simulink model "Power_Grid_Fault_Analysis_"  (R2019b)
settings: Solver=FixedStepAuto  StartTime=0.0  StopTime=0.2  RelTol=1e-3
InitFcn:
  | basekV = 23;
  | baseMVA = 100;
  | 
  | % base impedance
  | baseZ = (basekV)^2/baseMVA;
  | 
  | % nominal frequency
  | freq = 50;
libraries: powerlib x64, powerlib_meascontrol x17
(part 2 of 4)

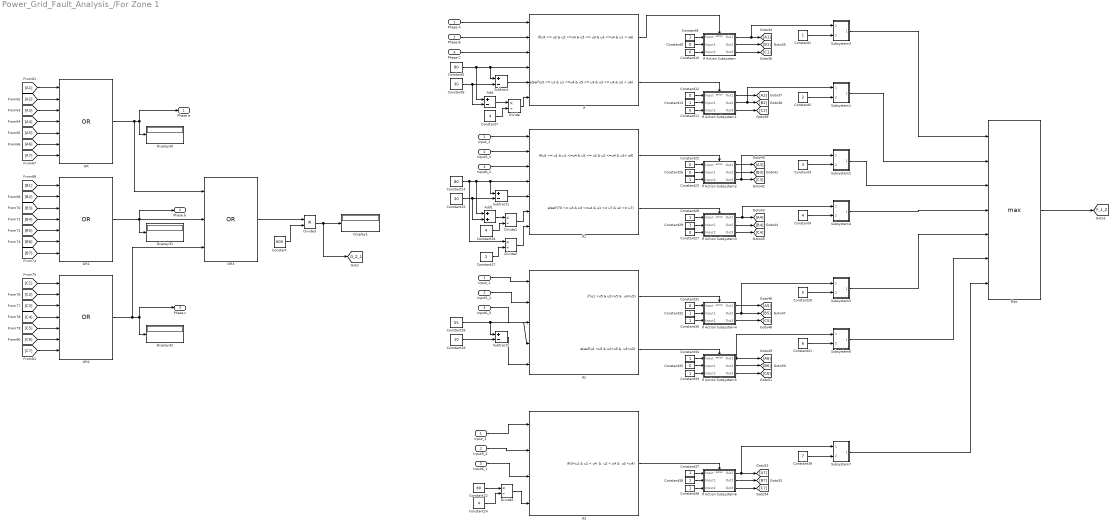
== system Power_Grid_Fault_Analysis_/For Zone 1 ==
  Phase A : Inport
  Phase B : Inport  Port=2
  Phase C : Inport  Port=3
  Add : Sum  Inputs=+-
  Add1 : Sum
  Constant : Constant  Value=600
  Constant{1,8,13,23,28..30,32..34,36..38} (13 alike) : Constant
  Constant{9..12,25..27,31,35} (9 alike) : Constant  Value=0
  Constant14 : Constant  Value=80
  Constant15 : Constant  Value=30
  Constant{4,7,16,24} (4 alike) : Constant  Value=4
  Constant17 : Constant  Value=2
  Constant18 : Constant  Value=55
  Constant19 : Constant  Value=10
  Constant2 : Constant  Value=2
  Constant20 : Constant  Value=5
  Constant21 : Constant  Value=6
  Constant22 : Constant  Value=80
  Constant3 : Constant  Value=3
  Constant39 : Constant  Value=7
  Constant5 : Constant  Value=80
  Constant6 : Constant  Value=30
  Display{1,30..32} (4 alike) : Display
      settings: Decimation=2
  Divide{,1..2,5} (4 alike) : Product  Inputs=*/  SaturateOnIntegerOverflow=on  RndMeth=Zero
  Divide3 : Product  Inputs=**  SaturateOnIntegerOverflow=on  RndMeth=Zero
  If : If  NumInputs=6  IfExpression=u5 <= u2 & u2 <=u4 & u5 <= u3 & u3 <=u4 & u1 < u6  ElseIfExpressions=u5 <= u1 & u1 <=u4 & u5 <= u3 & u3 <= u4 & u2 < u6  ShowElse=off
  If Action Subsystem : Subsystem  TreatAsAtomicUnit=on
  If Action Subsystem1 : Subsystem  TreatAsAtomicUnit=on
  If Action Subsystem2 : Subsystem  TreatAsAtomicUnit=on
  If Action Subsystem3 : Subsystem  TreatAsAtomicUnit=on
  If Action Subsystem4 : Subsystem  TreatAsAtomicUnit=on
  If Action Subsystem5 : Subsystem  TreatAsAtomicUnit=on
  If Action Subsystem6 : Subsystem  TreatAsAtomicUnit=on
  If1 : If  NumInputs=7  IfExpression=u5 <= u1 & u1 <=u4 & u5 <= u2 & u2 <=u4 & u3< u6  ElseIfExpressions=70 <= u3 & u3 <=u4 & u1 <= u7 & u2 <= u7  ShowElse=off
  If2 : If  NumInputs=5  IfExpression="u1 >u5 & u2<u5 &  u3<u5"  ElseIfExpressions="u1 <u5 & u2>u5 &  u3<u5"  ShowElse=off
  If3 : If  NumInputs=4  IfExpression="0<u1 & u1 < u4  &  u2 < u4 &  u3 <u4"  ShowElse=off
  Input5_1 : InportShadow  Port=2
  Input5_2 : InportShadow  Port=2
  Input5_3 : InportShadow  Port=2
  Input6_1 : InportShadow  Port=3
  Input6_2 : InportShadow  Port=3
  Input6_3 : InportShadow  Port=3
  Input_1 : InportShadow
  Input_2 : InportShadow
  Input_3 : InportShadow
  Max : MinMax  Function=max  Inputs=7
  OR : Logic  Operator=OR  Inputs=7  IconShape=distinctive  AllPortsSameDT=off  OutDataTypeStr=boolean
  OR1 : Logic  Operator=OR  Inputs=7  IconShape=distinctive  AllPortsSameDT=off  OutDataTypeStr=boolean
  OR2 : Logic  Operator=OR  Inputs=7  IconShape=distinctive  AllPortsSameDT=off  OutDataTypeStr=boolean
  OR3 : Logic  Operator=OR  Inputs=3  IconShape=distinctive  AllPortsSameDT=off  OutDataTypeStr=boolean
  Subsystem1 : Subsystem
  Subsystem2 : Subsystem
  Subsystem3 : Subsystem
  Subsystem4 : Subsystem
  Subsystem5 : Subsystem
  Subsystem6 : Subsystem
  Subsystem7 : Subsystem
  Subtract : Sum  Inputs=+-
  Subtract1 : Sum  Inputs=+-
  Subtract2 : Sum  Inputs=+-
  Phase a : Outport
  Phase b : Outport  Port=2
  Phase c : Outport  Port=3
  tag scope: D_Z_1=global, F_1_Z=global
  wires:
  If3/1 -> If Action Subsystem6/Action
  Constant5/1 -> Add/1, Subtract/1, If/4
  Constant14/1 -> Divide2/1, Subtract1/1, If1/4, Add1/1
  Constant33/1 -> If Action Subsystem5/3(Input2)
  Subtract/1 -> If/5
  Constant10/1 -> If Action Subsystem/3(Input2)
  Constant6/1 -> Add/2, Subtract/2
  Phase A/1 -> If/1
  Constant9/1 -> If Action Subsystem/2(Input1)
  If2/1 -> If Action Subsystem4/Action
  Constant30/1 -> If Action Subsystem4/3(Input2)
  Input_1/1 -> If2/1
  Input5_1/1 -> If2/2
  If Action Subsystem2/2(Out2) -> [B3]
  Phase B/1 -> If/2
  If2/2 -> If Action Subsystem5/Action
  If Action Subsystem/3(Out3) -> [C1]
  Constant15/1 -> Subtract1/2, Add1/2
  Input5_2/1 -> If3/2
  [A2] -> OR/2
  Input6_3/1 -> If2/3
  If Action Subsystem4/3(Out3) -> [C5]
  If1/1 -> If Action Subsystem2/Action
  Input6_2/1 -> If1/3
  Input_2/1 -> If1/1
  If Action Subsystem1/3(Out3) -> [C2]
  Phase C/1 -> If/3
  Constant24/1 -> Divide5/2
  Subtract2/1 -> If2/5
  Divide2/1 -> If1/7
  Constant18/1 -> Subtract2/1, If2/4
  Constant7/1 -> Divide/2
  Constant8/1 -> If Action Subsystem/1(Input)
  If Action Subsystem6/3(Out3) -> [C7]
  Constant16/1 -> Divide1/2
  If Action Subsystem1/1(Out1) -> [A2]
  Divide/1 -> If/6
  Subtract1/1 -> If1/5
  Constant28/1 -> If Action Subsystem3/1(Input)
  Add1/1 -> Divide1/1
  Constant19/1 -> Subtract2/2
  If/2 -> If Action Subsystem1/Action
  Constant38/1 -> If Action Subsystem6/2(Input1)
  Constant13/1 -> If Action Subsystem1/2(Input1)
  Constant12/1 -> If Action Subsystem1/1(Input)
  If Action Subsystem3/2(Out2) -> [B4]
  Constant17/1 -> Divide2/2
  Constant32/1 -> If Action Subsystem4/2(Input1)
  Constant11/1 -> If Action Subsystem1/3(Input2)
  [A3] -> OR/3
  Constant29/1 -> If Action Subsystem3/2(Input1)
  Constant26/1 -> If Action Subsystem2/2(Input1)
  Add/1 -> Divide/1
  If Action Subsystem3/1(Out1) -> Subsystem4/1(In1), [A4]
  Divide1/1 -> If1/6
  Input_3/1 -> If3/1
  Constant34/1 -> If Action Subsystem5/1(Input)
  Constant27/1 -> If Action Subsystem3/3(Input2)
  Constant25/1 -> If Action Subsystem2/1(Input)
  If/1 -> If Action Subsystem/Action
  Constant22/1 -> Divide5/1
  Constant37/1 -> If Action Subsystem6/1(Input)
  If1/2 -> If Action Subsystem3/Action
  [C4] -> OR2/4
  Divide5/1 -> If3/4
  If Action Subsystem/2(Out2) -> [B1]
  [A1] -> OR/1
  [B5] -> OR1/5
  [B7] -> OR1/7
  [A4] -> OR/4
  If Action Subsystem6/2(Out2) -> [B7]
  [B3] -> OR1/3
  [B6] -> OR1/6
  [B2] -> OR1/2
  If Action Subsystem5/2(Out2) -> [B6]
  If Action Subsystem5/3(Out3) -> [C6]
  [A5] -> OR/5
  [C5] -> OR2/5
  [C1] -> OR2/1
  Constant23/1 -> If Action Subsystem2/3(Input2)
  Constant35/1 -> If Action Subsystem5/2(Input1)
  Input6_1/1 -> If3/3
  [A7] -> OR/7
  [C7] -> OR2/7
  Constant36/1 -> If Action Subsystem6/3(Input2)
  If Action Subsystem4/1(Out1) -> [A5]
  [C3] -> OR2/3
  [B1] -> OR1/1
  [A6] -> OR/6
  Constant31/1 -> If Action Subsystem4/1(Input)
  If Action Subsystem2/1(Out1) -> [A3]
  [C2] -> OR2/2
  [B4] -> OR1/4
  [C6] -> OR2/6
  Input5_3/1 -> If1/2
  Divide3/1 -> [D_Z_1], Display1/1
  OR3/1 -> Divide3/1
  OR2/1 -> OR3/3, Phase c/1, Display32/1
  OR1/1 -> OR3/2, Phase b/1, Display31/1
  Constant/1 -> Divide3/2
  OR/1 -> OR3/1, Phase a/1, Display30/1
  If Action Subsystem/1(Out1) -> Subsystem3/1(In1), [A1]
  Constant1/1 -> Subsystem3/2(In2)
  If Action Subsystem1/2(Out2) -> Subsystem1/1(In1), [B2]
  Constant2/1 -> Subsystem1/2(In2)
  If Action Subsystem2/3(Out3) -> Subsystem2/1(In1), [C3]
  Constant3/1 -> Subsystem2/2(In2)
  Constant4/1 -> Subsystem4/2(In2)
  If Action Subsystem3/3(Out3) -> [C4]
  Constant20/1 -> Subsystem5/2(In2)
  If Action Subsystem4/2(Out2) -> Subsystem5/1(In1), [B5]
  Constant21/1 -> Subsystem6/2(In2)
  If Action Subsystem5/1(Out1) -> Subsystem6/1(In1), [A6]
  Constant39/1 -> Subsystem7/2(In2)
  If Action Subsystem6/1(Out1) -> Subsystem7/1(In1), [A7]
  Subsystem3/1(Output) -> Max/1
  Subsystem1/1(Output) -> Max/2
  Subsystem2/1(Output) -> Max/3
  Subsystem4/1(Output) -> Max/4
  Subsystem5/1(Output) -> Max/5
  Subsystem6/1(Output) -> Max/6
  Subsystem7/1(Output) -> Max/7
  Max/1 -> [F_1_Z]

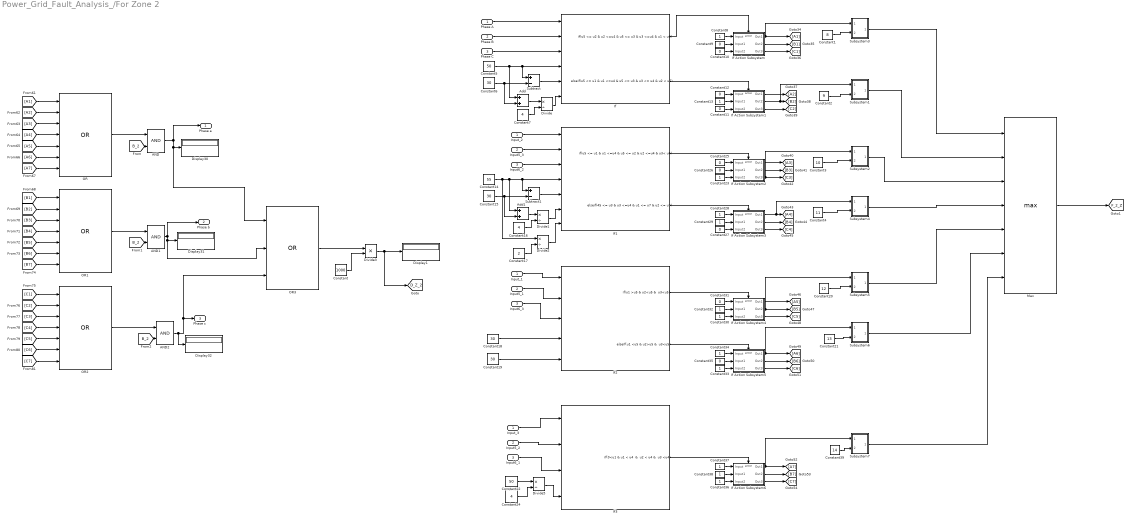
== system Power_Grid_Fault_Analysis_/For Zone 2 ==
  Phase A : Inport
  Phase B : Inport  Port=2
  Phase C : Inport  Port=3
  AND : Logic  IconShape=distinctive  AllPortsSameDT=off  OutDataTypeStr=boolean
  AND1 : Logic  IconShape=distinctive  AllPortsSameDT=off  OutDataTypeStr=boolean
  AND2 : Logic  IconShape=distinctive  AllPortsSameDT=off  OutDataTypeStr=boolean
  Add : Sum
  Add1 : Sum
  Constant : Constant  Value=1000
  Constant1 : Constant  Value=8
  Constant{9..12,25..27,31,35} (9 alike) : Constant  Value=0
  Constant{8,13,23,28..30,32..34,36..38} (12 alike) : Constant
  Constant14 : Constant  Value=55
  Constant{6,15,18..19} (4 alike) : Constant  Value=30
  Constant16 : Constant  Value=4
  Constant17 : Constant  Value=2
  Constant2 : Constant  Value=9
  Constant20 : Constant  Value=12
  Constant21 : Constant  Value=13
  Constant22 : Constant  Value=50
  Constant24 : Constant  Value=4
  Constant3 : Constant  Value=10
  Constant39 : Constant  Value=14
  Constant4 : Constant  Value=11
  Constant5 : Constant  Value=50
  Constant7 : Constant  Value=4
  Display{1,30..32} (4 alike) : Display
      settings: Decimation=2
  Divide{,1..2,5} (4 alike) : Product  Inputs=*/  SaturateOnIntegerOverflow=on  RndMeth=Zero
  Divide3 : Product  Inputs=**  SaturateOnIntegerOverflow=on  RndMeth=Zero
  If : If  NumInputs=6  IfExpression=u5 <= u2 & u2 <=u4 & u5 <= u3 & u3 <=u4 & u1 < u6  ElseIfExpressions=u5 <= u1 & u1 <=u4 & u5 <= u3 & u3 <= u4 & u2 < u6  ShowElse=off
  If Action Subsystem : Subsystem  TreatAsAtomicUnit=on
  If Action Subsystem1 : Subsystem  TreatAsAtomicUnit=on
  If Action Subsystem2 : Subsystem  TreatAsAtomicUnit=on
  If Action Subsystem3 : Subsystem  TreatAsAtomicUnit=on
  If Action Subsystem4 : Subsystem  TreatAsAtomicUnit=on
  If Action Subsystem5 : Subsystem  TreatAsAtomicUnit=on
  If Action Subsystem6 : Subsystem  TreatAsAtomicUnit=on
  If1 : If  NumInputs=7  IfExpression=u5 <= u1 & u1 <=u4 & u5 <= u2 & u2 <=u4 & u3< u6  ElseIfExpressions=45 <= u3 & u3 <=u4 & u1 <= u7 & u2 <= u7  ShowElse=off
  If2 : If  NumInputs=5  IfExpression="u1 >u5 & u2<u5 &  u3<u5"  ElseIfExpressions="u1 <u5 & u2>u5 &  u3<u5"  ShowElse=off
  If3 : If  NumInputs=4  IfExpression="0<u1 & u1 < u4  &  u2 < u4 &  u3 <u4"  ShowElse=off
  Input5_1 : InportShadow  Port=2
  Input5_2 : InportShadow  Port=2
  Input5_3 : InportShadow  Port=2
  Input6_1 : InportShadow  Port=3
  Input6_2 : InportShadow  Port=3
  Input6_3 : InportShadow  Port=3
  Input_1 : InportShadow
  Input_2 : InportShadow
  Input_3 : InportShadow
  Max : MinMax  Function=max  Inputs=7
  OR : Logic  Operator=OR  Inputs=7  IconShape=distinctive  AllPortsSameDT=off  OutDataTypeStr=boolean
  OR1 : Logic  Operator=OR  Inputs=7  IconShape=distinctive  AllPortsSameDT=off  OutDataTypeStr=boolean
  OR2 : Logic  Operator=OR  Inputs=7  IconShape=distinctive  AllPortsSameDT=off  OutDataTypeStr=boolean
  OR3 : Logic  Operator=OR  Inputs=3  IconShape=distinctive  AllPortsSameDT=off  OutDataTypeStr=boolean
  Subsystem1 : Subsystem
  Subsystem2 : Subsystem
  Subsystem3 : Subsystem
  Subsystem4 : Subsystem
  Subsystem5 : Subsystem
  Subsystem6 : Subsystem
  Subsystem7 : Subsystem
  Subtract : Sum  Inputs=+-
  Subtract1 : Sum  Inputs=+-
  Phase a : Outport
  Phase b : Outport  Port=2
  Phase c : Outport  Port=3
  tag scope: D_Z_2=global, F_2_Z=global
  wires:
  If3/1 -> If Action Subsystem6/Action
  Constant5/1 -> Add/1, Subtract/1, If/4
  Constant14/1 -> Divide2/1, Subtract1/1, If1/4, Add1/1
  Constant33/1 -> If Action Subsystem5/3(Input2)
  Subtract/1 -> If/5
  Constant10/1 -> If Action Subsystem/3(Input2)
  Constant6/1 -> Add/2, Subtract/2
  Phase A/1 -> If/1
  Constant9/1 -> If Action Subsystem/2(Input1)
  If2/1 -> If Action Subsystem4/Action
  Constant30/1 -> If Action Subsystem4/3(Input2)
  Input_1/1 -> If2/1
  Input5_1/1 -> If2/2
  If Action Subsystem2/2(Out2) -> [B3]
  Phase B/1 -> If/2
  If2/2 -> If Action Subsystem5/Action
  If Action Subsystem/3(Out3) -> [C1]
  Constant15/1 -> Subtract1/2, Add1/2
  Input5_2/1 -> If3/2
  [A2] -> OR/2
  Input6_3/1 -> If2/3
  If Action Subsystem4/3(Out3) -> [C5]
  If1/1 -> If Action Subsystem2/Action
  Input6_2/1 -> If1/3
  Input_2/1 -> If1/1
  If Action Subsystem1/3(Out3) -> [C2]
  Phase C/1 -> If/3
  Constant24/1 -> Divide5/2
  Constant19/1 -> If2/5
  Divide2/1 -> If1/7
  Constant18/1 -> If2/4
  Constant7/1 -> Divide/2
  Constant8/1 -> If Action Subsystem/1(Input)
  If Action Subsystem6/3(Out3) -> [C7]
  Constant16/1 -> Divide1/2
  If Action Subsystem1/1(Out1) -> [A2]
  Divide/1 -> If/6
  Subtract1/1 -> If1/5
  Constant28/1 -> If Action Subsystem3/1(Input)
  Add1/1 -> Divide1/1
  If/2 -> If Action Subsystem1/Action
  Constant38/1 -> If Action Subsystem6/2(Input1)
  Constant13/1 -> If Action Subsystem1/2(Input1)
  Constant12/1 -> If Action Subsystem1/1(Input)
  If Action Subsystem3/2(Out2) -> [B4]
  Constant17/1 -> Divide2/2
  Constant32/1 -> If Action Subsystem4/2(Input1)
  Constant11/1 -> If Action Subsystem1/3(Input2)
  [A3] -> OR/3
  Constant29/1 -> If Action Subsystem3/2(Input1)
  Constant26/1 -> If Action Subsystem2/2(Input1)
  Add/1 -> Divide/1
  If Action Subsystem3/1(Out1) -> Subsystem4/1(In1), [A4]
  Divide1/1 -> If1/6
  Input_3/1 -> If3/1
  Constant34/1 -> If Action Subsystem5/1(Input)
  Constant27/1 -> If Action Subsystem3/3(Input2)
  Constant25/1 -> If Action Subsystem2/1(Input)
  If/1 -> If Action Subsystem/Action
  Constant22/1 -> Divide5/1
  Constant37/1 -> If Action Subsystem6/1(Input)
  If1/2 -> If Action Subsystem3/Action
  [C4] -> OR2/4
  Divide5/1 -> If3/4
  If Action Subsystem/2(Out2) -> [B1]
  [A1] -> OR/1
  [B5] -> OR1/5
  [B7] -> OR1/7
  [A4] -> OR/4
  If Action Subsystem6/2(Out2) -> [B7]
  [B3] -> OR1/3
  [B6] -> OR1/6
  [B2] -> OR1/2
  If Action Subsystem5/2(Out2) -> [B6]
  If Action Subsystem5/3(Out3) -> [C6]
  [A5] -> OR/5
  [C5] -> OR2/5
  [C1] -> OR2/1
  Constant23/1 -> If Action Subsystem2/3(Input2)
  Constant35/1 -> If Action Subsystem5/2(Input1)
  Input6_1/1 -> If3/3
  [A7] -> OR/7
  [C7] -> OR2/7
  Constant36/1 -> If Action Subsystem6/3(Input2)
  If Action Subsystem4/1(Out1) -> [A5]
  [C3] -> OR2/3
  [B1] -> OR1/1
  [A6] -> OR/6
  Constant31/1 -> If Action Subsystem4/1(Input)
  If Action Subsystem2/1(Out1) -> [A3]
  [C2] -> OR2/2
  [B4] -> OR1/4
  [C6] -> OR2/6
  Input5_3/1 -> If1/2
  Divide3/1 -> [D_Z_2], Display1/1
  OR3/1 -> Divide3/1
  Constant/1 -> Divide3/2
  [B_2] -> AND/2
  OR/1 -> AND/1
  AND/1 -> Phase a/1, OR3/1, Display30/1
  [B_2] -> AND1/2
  OR1/1 -> AND1/1
  AND1/1 -> Phase b/1, OR3/2, Display31/1
  [B_2] -> AND2/2
  OR2/1 -> AND2/1
  AND2/1 -> Display32/1, OR3/3, Phase c/1
  If Action Subsystem6/1(Out1) -> Subsystem7/1(In1), [A7]
  If Action Subsystem/1(Out1) -> Subsystem3/1(In1), [A1]
  If Action Subsystem1/2(Out2) -> Subsystem1/1(In1), [B2]
  Constant20/1 -> Subsystem5/2(In2)
  Constant21/1 -> Subsystem6/2(In2)
  Constant4/1 -> Subsystem4/2(In2)
  Constant39/1 -> Subsystem7/2(In2)
  If Action Subsystem3/3(Out3) -> [C4]
  If Action Subsystem2/3(Out3) -> Subsystem2/1(In1), [C3]
  If Action Subsystem5/1(Out1) -> Subsystem6/1(In1), [A6]
  Constant2/1 -> Subsystem1/2(In2)
  Constant1/1 -> Subsystem3/2(In2)
  If Action Subsystem4/2(Out2) -> Subsystem5/1(In1), [B5]
  Constant3/1 -> Subsystem2/2(In2)
  Subsystem1/1(Output) -> Max/2
  Max/1 -> [F_2_Z]
  Subsystem7/1(Output) -> Max/7
  Subsystem6/1(Output) -> Max/6
  Subsystem5/1(Output) -> Max/5
  Subsystem4/1(Output) -> Max/4
  Subsystem2/1(Output) -> Max/3
  Subsystem3/1(Output) -> Max/1

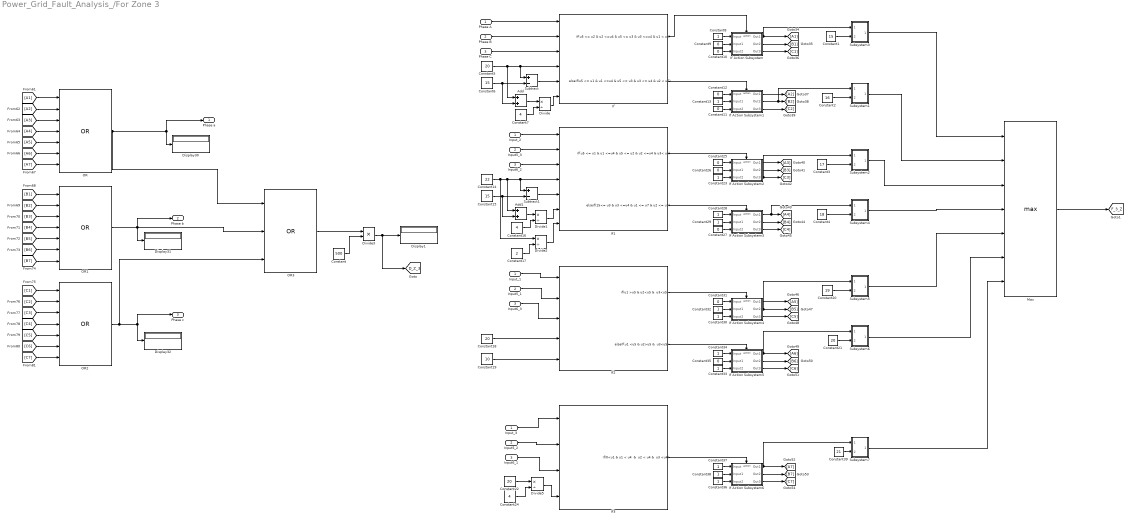
== system Power_Grid_Fault_Analysis_/For Zone 3 ==
  Phase A : Inport
  Phase B : Inport  Port=2
  Phase C : Inport  Port=3
  Add : Sum
  Add1 : Sum
  Constant : Constant  Value=500
  Constant1 : Constant  Value=15
  Constant{9..12,25..27,31,35} (9 alike) : Constant  Value=0
  Constant{8,13,23,28..30,32..34,36..38} (12 alike) : Constant
  Constant14 : Constant  Value=22
  Constant15 : Constant  Value=15
  Constant16 : Constant  Value=4
  Constant17 : Constant  Value=2
  Constant{5,18,21..22} (4 alike) : Constant  Value=20
  Constant19 : Constant  Value=10
  Constant2 : Constant  Value=16
  Constant20 : Constant  Value=19
  Constant24 : Constant  Value=4
  Constant3 : Constant  Value=17
  Constant39 : Constant  Value=21
  Constant4 : Constant  Value=18
  Constant6 : Constant  Value=15
  Constant7 : Constant  Value=4
  Display{1,30..32} (4 alike) : Display
      settings: Decimation=2
  Divide{,1..2,5} (4 alike) : Product  Inputs=*/  SaturateOnIntegerOverflow=on  RndMeth=Zero
  Divide3 : Product  Inputs=**  SaturateOnIntegerOverflow=on  RndMeth=Zero
  If : If  NumInputs=6  IfExpression=u5 <= u2 & u2 <=u4 & u5 <= u3 & u3 <=u4 & u1 < u6  ElseIfExpressions=u5 <= u1 & u1 <=u4 & u5 <= u3 & u3 <= u4 & u2 < u6  ShowElse=off
  If Action Subsystem : Subsystem  TreatAsAtomicUnit=on
  If Action Subsystem1 : Subsystem  TreatAsAtomicUnit=on
  If Action Subsystem2 : Subsystem  TreatAsAtomicUnit=on
  If Action Subsystem3 : Subsystem  TreatAsAtomicUnit=on
  If Action Subsystem4 : Subsystem  TreatAsAtomicUnit=on
  If Action Subsystem5 : Subsystem  TreatAsAtomicUnit=on
  If Action Subsystem6 : Subsystem  TreatAsAtomicUnit=on
  If1 : If  NumInputs=7  IfExpression=u5 <= u1 & u1 <=u4 & u5 <= u2 & u2 <=u4 & u3< u6  ElseIfExpressions=15<= u3 & u3 <=u4 & u1 <= u7 & u2 <= u7  ShowElse=off
  If2 : If  NumInputs=5  IfExpression="u1 >u5 & u2<u5 &  u3<u5"  ElseIfExpressions="u1 <u5 & u2>u5 &  u3<u5"  ShowElse=off
  If3 : If  NumInputs=4  IfExpression="0<u1 & u1 < u4  &  u2 < u4 &  u3 <u4"  ShowElse=off
  Input5_1 : InportShadow  Port=2
  Input5_2 : InportShadow  Port=2
  Input5_3 : InportShadow  Port=2
  Input6_1 : InportShadow  Port=3
  Input6_2 : InportShadow  Port=3
  Input6_3 : InportShadow  Port=3
  Input_1 : InportShadow
  Input_2 : InportShadow
  Input_3 : InportShadow
  Max : MinMax  Function=max  Inputs=7
  OR : Logic  Operator=OR  Inputs=7  IconShape=distinctive  AllPortsSameDT=off  OutDataTypeStr=boolean
  OR1 : Logic  Operator=OR  Inputs=7  IconShape=distinctive  AllPortsSameDT=off  OutDataTypeStr=boolean
  OR2 : Logic  Operator=OR  Inputs=7  IconShape=distinctive  AllPortsSameDT=off  OutDataTypeStr=boolean
  OR3 : Logic  Operator=OR  Inputs=3  IconShape=distinctive  AllPortsSameDT=off  OutDataTypeStr=boolean
  Subsystem1 : Subsystem
  Subsystem2 : Subsystem
  Subsystem3 : Subsystem
  Subsystem4 : Subsystem
  Subsystem5 : Subsystem
  Subsystem6 : Subsystem
  Subsystem7 : Subsystem
  Subtract : Sum  Inputs=+-
  Subtract1 : Sum  Inputs=+-
  Phase a : Outport
  Phase b : Outport  Port=2
  Phase c : Outport  Port=3
  tag scope: D_Z_3=global, F_3_Z=global
  wires:
  If3/1 -> If Action Subsystem6/Action
  Constant5/1 -> Add/1, Subtract/1, If/4
  Constant14/1 -> Divide2/1, Subtract1/1, If1/4, Add1/1
  Constant33/1 -> If Action Subsystem5/3(Input2)
  Subtract/1 -> If/5
  Constant10/1 -> If Action Subsystem/3(Input2)
  Constant6/1 -> Add/2, Subtract/2
  Phase A/1 -> If/1
  Constant9/1 -> If Action Subsystem/2(Input1)
  If2/1 -> If Action Subsystem4/Action
  Constant30/1 -> If Action Subsystem4/3(Input2)
  Input_1/1 -> If2/1
  Input5_1/1 -> If2/2
  If Action Subsystem2/2(Out2) -> [B3]
  Phase B/1 -> If/2
  If2/2 -> If Action Subsystem5/Action
  If Action Subsystem/3(Out3) -> [C1]
  Constant15/1 -> Subtract1/2, Add1/2
  Input5_2/1 -> If3/2
  [A2] -> OR/2
  Input6_3/1 -> If2/3
  If Action Subsystem4/3(Out3) -> [C5]
  If1/1 -> If Action Subsystem2/Action
  Input6_2/1 -> If1/3
  Input_2/1 -> If1/1
  If Action Subsystem1/3(Out3) -> [C2]
  Phase C/1 -> If/3
  Constant24/1 -> Divide5/2
  Constant19/1 -> If2/5
  Divide2/1 -> If1/7
  Constant18/1 -> If2/4
  Constant7/1 -> Divide/2
  Constant8/1 -> If Action Subsystem/1(Input)
  If Action Subsystem6/3(Out3) -> [C7]
  Constant16/1 -> Divide1/2
  If Action Subsystem1/1(Out1) -> [A2]
  Divide/1 -> If/6
  Subtract1/1 -> If1/5
  Constant28/1 -> If Action Subsystem3/1(Input)
  Add1/1 -> Divide1/1
  If/2 -> If Action Subsystem1/Action
  Constant38/1 -> If Action Subsystem6/2(Input1)
  Constant13/1 -> If Action Subsystem1/2(Input1)
  Constant12/1 -> If Action Subsystem1/1(Input)
  If Action Subsystem3/2(Out2) -> [B4]
  Constant17/1 -> Divide2/2
  Constant32/1 -> If Action Subsystem4/2(Input1)
  Constant11/1 -> If Action Subsystem1/3(Input2)
  [A3] -> OR/3
  Constant29/1 -> If Action Subsystem3/2(Input1)
  Constant26/1 -> If Action Subsystem2/2(Input1)
  Add/1 -> Divide/1
  Divide1/1 -> If1/6
  Input_3/1 -> If3/1
  Constant34/1 -> If Action Subsystem5/1(Input)
  Constant27/1 -> If Action Subsystem3/3(Input2)
  Constant25/1 -> If Action Subsystem2/1(Input)
  If/1 -> If Action Subsystem/Action
  Constant22/1 -> Divide5/1
  Constant37/1 -> If Action Subsystem6/1(Input)
  If1/2 -> If Action Subsystem3/Action
  [C4] -> OR2/4
  Divide5/1 -> If3/4
  If Action Subsystem/2(Out2) -> [B1]
  [A1] -> OR/1
  [B5] -> OR1/5
  [B7] -> OR1/7
  [A4] -> OR/4
  If Action Subsystem6/2(Out2) -> [B7]
  [B3] -> OR1/3
  [B6] -> OR1/6
  [B2] -> OR1/2
  If Action Subsystem5/2(Out2) -> [B6]
  If Action Subsystem5/3(Out3) -> [C6]
  [A5] -> OR/5
  [C5] -> OR2/5
  [C1] -> OR2/1
  Constant23/1 -> If Action Subsystem2/3(Input2)
  Constant35/1 -> If Action Subsystem5/2(Input1)
  Input6_1/1 -> If3/3
  [A7] -> OR/7
  [C7] -> OR2/7
  Constant36/1 -> If Action Subsystem6/3(Input2)
  If Action Subsystem4/1(Out1) -> [A5]
  [C3] -> OR2/3
  [B1] -> OR1/1
  [A6] -> OR/6
  Constant31/1 -> If Action Subsystem4/1(Input)
  If Action Subsystem3/3(Out3) -> [C4]
  If Action Subsystem2/1(Out1) -> [A3]
  [C2] -> OR2/2
  [B4] -> OR1/4
  [C6] -> OR2/6
  Input5_3/1 -> If1/2
  Divide3/1 -> [D_Z_3], Display1/1
  OR3/1 -> Divide3/1
  OR2/1 -> OR3/3, Phase c/1, Display32/1
  OR1/1 -> OR3/2, Phase b/1, Display31/1
  Constant/1 -> Divide3/2
  OR/1 -> Display30/1, Phase a/1, OR3/1
  If Action Subsystem/1(Out1) -> Subsystem3/1(In1), [A1]
  If Action Subsystem6/1(Out1) -> Subsystem7/1(In1), [A7]
  If Action Subsystem4/2(Out2) -> Subsystem5/1(In1), [B5]
  If Action Subsystem2/3(Out3) -> Subsystem2/1(In1), [C3]
  Constant1/1 -> Subsystem3/2(In2)
  Constant20/1 -> Subsystem5/2(In2)
  Constant4/1 -> Subsystem4/2(In2)
  Constant3/1 -> Subsystem2/2(In2)
  Constant21/1 -> Subsystem6/2(In2)
  Constant39/1 -> Subsystem7/2(In2)
  Constant2/1 -> Subsystem1/2(In2)
  If Action Subsystem1/2(Out2) -> Subsystem1/1(In1), [B2]
  If Action Subsystem5/1(Out1) -> Subsystem6/1(In1), [A6]
  If Action Subsystem3/1(Out1) -> Subsystem4/1(In1), [A4]
  Subsystem1/1(Output) -> Max/2
  Max/1 -> [F_3_Z]
  Subsystem7/1(Output) -> Max/7
  Subsystem6/1(Output) -> Max/6
  Subsystem5/1(Output) -> Max/5
  Subsystem4/1(Output) -> Max/4
  Subsystem2/1(Output) -> Max/3
  Subsystem3/1(Output) -> Max/1

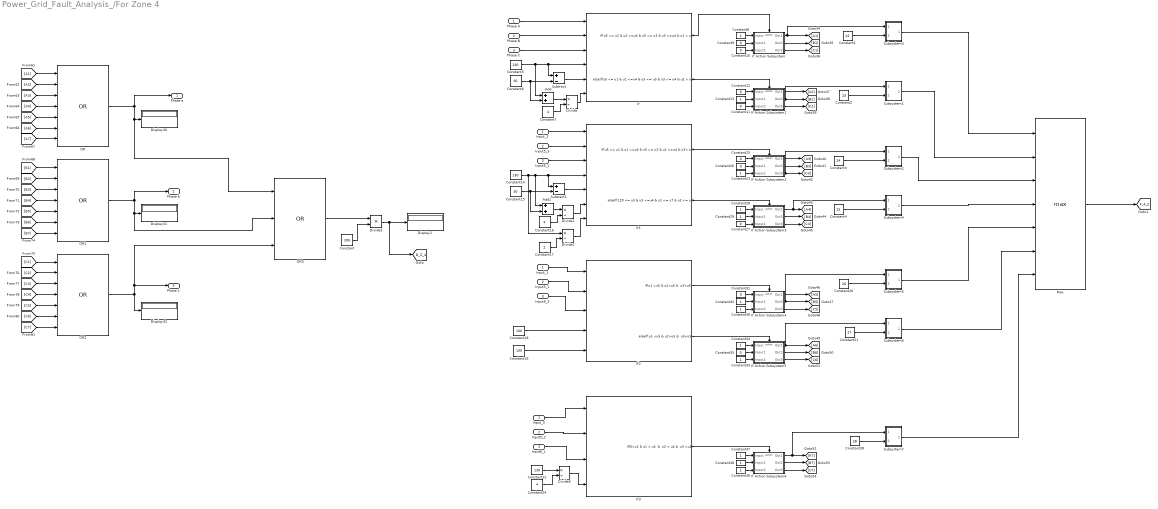
== system Power_Grid_Fault_Analysis_/For Zone 4 ==
  Phase A : Inport
  Phase B : Inport  Port=2
  Phase C : Inport  Port=3
  Add : Sum
  Add1 : Sum
  Constant : Constant  Value=200
  Constant1 : Constant  Value=22
  Constant{9..12,25..27,31,35} (9 alike) : Constant  Value=0
  Constant{8,13,23,28..30,32..34,36..38} (12 alike) : Constant
  Constant14 : Constant  Value=130
  Constant15 : Constant  Value=30
  Constant16 : Constant  Value=4
  Constant17 : Constant  Value=2
  Constant18 : Constant  Value=100
  Constant19 : Constant  Value=100
  Constant2 : Constant  Value=23
  Constant20 : Constant  Value=26
  Constant21 : Constant  Value=27
  Constant22 : Constant  Value=130
  Constant24 : Constant  Value=4
  Constant3 : Constant  Value=24
  Constant39 : Constant  Value=28
  Constant4 : Constant  Value=25
  Constant5 : Constant  Value=130
  Constant6 : Constant  Value=30
  Constant7 : Constant  Value=4
  Display{1,30..32} (4 alike) : Display
      settings: Decimation=2
  Divide{,1..2,5} (4 alike) : Product  Inputs=*/  SaturateOnIntegerOverflow=on  RndMeth=Zero
  Divide3 : Product  Inputs=**  SaturateOnIntegerOverflow=on  RndMeth=Zero
  If : If  NumInputs=6  IfExpression=u5 <= u2 & u2 <=u4 & u5 <= u3 & u3 <=u4 & u1 < u6  ElseIfExpressions=u5 <= u1 & u1 <=u4 & u5 <= u3 & u3 <= u4 & u2 < u6  ShowElse=off
  If Action Subsystem : Subsystem  TreatAsAtomicUnit=on
  If Action Subsystem1 : Subsystem  TreatAsAtomicUnit=on
  If Action Subsystem2 : Subsystem  TreatAsAtomicUnit=on
  If Action Subsystem3 : Subsystem  TreatAsAtomicUnit=on
  If Action Subsystem4 : Subsystem  TreatAsAtomicUnit=on
  If Action Subsystem5 : Subsystem  TreatAsAtomicUnit=on
  If Action Subsystem6 : Subsystem  TreatAsAtomicUnit=on
  If1 : If  NumInputs=7  IfExpression=u5 <= u1 & u1 <=u4 & u5 <= u2 & u2 <=u4 & u3< u6  ElseIfExpressions=120 <= u3 & u3 <=u4 & u1 <= u7 & u2 <= u7  ShowElse=off
  If2 : If  NumInputs=5  IfExpression="u1 >u5 & u2<u5 &  u3<u5"  ElseIfExpressions="u1 <u5 & u2>u5 &  u3<u5"  ShowElse=off
  If3 : If  NumInputs=4  IfExpression="0<u1 & u1 < u4  &  u2 < u4 &  u3 <u4"  ShowElse=off
  Input5_1 : InportShadow  Port=2
  Input5_2 : InportShadow  Port=2
  Input5_3 : InportShadow  Port=2
  Input6_1 : InportShadow  Port=3
  Input6_2 : InportShadow  Port=3
  Input6_3 : InportShadow  Port=3
  Input_1 : InportShadow
  Input_2 : InportShadow
  Input_3 : InportShadow
  Max : MinMax  Function=max  Inputs=7
  OR : Logic  Operator=OR  Inputs=7  IconShape=distinctive  AllPortsSameDT=off  OutDataTypeStr=boolean
  OR1 : Logic  Operator=OR  Inputs=7  IconShape=distinctive  AllPortsSameDT=off  OutDataTypeStr=boolean
  OR2 : Logic  Operator=OR  Inputs=7  IconShape=distinctive  AllPortsSameDT=off  OutDataTypeStr=boolean
  OR3 : Logic  Operator=OR  Inputs=3  IconShape=distinctive  AllPortsSameDT=off  OutDataTypeStr=boolean
  Subsystem1 : Subsystem
  Subsystem2 : Subsystem
  Subsystem3 : Subsystem
  Subsystem4 : Subsystem
  Subsystem5 : Subsystem
  Subsystem6 : Subsystem
  Subsystem7 : Subsystem
  Subtract : Sum  Inputs=+-
  Subtract1 : Sum  Inputs=+-
  Phase a : Outport
  Phase b : Outport  Port=2
  Phase c : Outport  Port=3
  tag scope: D_Z_4=global, F_4_Z=global
  wires:
  Subtract/1 -> If/5
  Constant19/1 -> If2/5
  If Action Subsystem/2(Out2) -> [B1]
  [C3] -> OR2/3
  [C6] -> OR2/6
  Constant12/1 -> If Action Subsystem1/1(Input)
  Input5_2/1 -> If3/2
  Input5_1/1 -> If2/2
  Constant33/1 -> If Action Subsystem5/3(Input2)
  If2/1 -> If Action Subsystem4/Action
  Phase A/1 -> If/1
  Constant9/1 -> If Action Subsystem/2(Input1)
  Phase B/1 -> If/2
  Constant15/1 -> Subtract1/2, Add1/2
  Input_1/1 -> If2/1
  If Action Subsystem3/3(Out3) -> [C4]
  Constant6/1 -> Add/2, Subtract/2
  Constant10/1 -> If Action Subsystem/3(Input2)
  If3/1 -> If Action Subsystem6/Action
  If Action Subsystem5/3(Out3) -> [C6]
  Constant30/1 -> If Action Subsystem4/3(Input2)
  Input5_3/1 -> If1/2
  [B1] -> OR1/1
  [C7] -> OR2/7
  [A5] -> OR/5
  Add1/1 -> Divide1/1
  [B2] -> OR1/2
  If/1 -> If Action Subsystem/Action
  [B6] -> OR1/6
  If Action Subsystem6/3(Out3) -> [C7]
  [B3] -> OR1/3
  If Action Subsystem3/2(Out2) -> [B4]
  Input6_3/1 -> If2/3
  If Action Subsystem4/3(Out3) -> [C5]
  Constant38/1 -> If Action Subsystem6/2(Input1)
  [B7] -> OR1/7
  [B5] -> OR1/5
  [C4] -> OR2/4
  Input_3/1 -> If3/1
  Divide/1 -> If/6
  If2/2 -> If Action Subsystem5/Action
  If Action Subsystem6/2(Out2) -> [B7]
  If1/2 -> If Action Subsystem3/Action
  Constant37/1 -> If Action Subsystem6/1(Input)
  Constant25/1 -> If Action Subsystem2/1(Input)
  Constant11/1 -> If Action Subsystem1/3(Input2)
  Constant17/1 -> Divide2/2
  Constant27/1 -> If Action Subsystem3/3(Input2)
  Constant26/1 -> If Action Subsystem2/2(Input1)
  Constant34/1 -> If Action Subsystem5/1(Input)
  Constant5/1 -> Add/1, Subtract/1, If/4
  Constant24/1 -> Divide5/2
  If/2 -> If Action Subsystem1/Action
  Constant8/1 -> If Action Subsystem/1(Input)
  Subtract1/1 -> If1/5
  If Action Subsystem1/1(Out1) -> [A2]
  Constant22/1 -> Divide5/1
  Divide2/1 -> If1/7
  If Action Subsystem1/3(Out3) -> [C2]
  Divide1/1 -> If1/6
  Input6_2/1 -> If1/3
  Phase C/1 -> If/3
  [A2] -> OR/2
  OR/1 -> Phase a/1, OR3/1, Display30/1
  [A4] -> OR/4
  OR1/1 -> Phase b/1, OR3/2, Display31/1
  If1/1 -> If Action Subsystem2/Action
  Constant32/1 -> If Action Subsystem4/2(Input1)
  If Action Subsystem2/2(Out2) -> [B3]
  If Action Subsystem5/2(Out2) -> [B6]
  Constant31/1 -> If Action Subsystem4/1(Input)
  [A3] -> OR/3
  Constant13/1 -> If Action Subsystem1/2(Input1)
  [A7] -> OR/7
  If Action Subsystem2/1(Out1) -> [A3]
  [A6] -> OR/6
  [B4] -> OR1/4
  Divide5/1 -> If3/4
  [C2] -> OR2/2
  Add/1 -> Divide/1
  Constant36/1 -> If Action Subsystem6/3(Input2)
  Constant35/1 -> If Action Subsystem5/2(Input1)
  Constant18/1 -> If2/4
  OR2/1 -> OR3/3, Phase c/1, Display32/1
  [C1] -> OR2/1
  [C5] -> OR2/5
  If Action Subsystem/3(Out3) -> [C1]
  Constant14/1 -> Divide2/1, Subtract1/1, If1/4, Add1/1
  Input_2/1 -> If1/1
  If Action Subsystem4/1(Out1) -> [A5]
  Input6_1/1 -> If3/3
  Constant7/1 -> Divide/2
  Constant29/1 -> If Action Subsystem3/2(Input1)
  [A1] -> OR/1
  Constant16/1 -> Divide1/2
  Constant28/1 -> If Action Subsystem3/1(Input)
  Constant23/1 -> If Action Subsystem2/3(Input2)
  OR3/1 -> Divide3/1
  Constant/1 -> Divide3/2
  Divide3/1 -> [D_Z_4], Display1/1
  If Action Subsystem/1(Out1) -> Subsystem3/1(In1), [A1]
  If Action Subsystem6/1(Out1) -> Subsystem7/1(In1), [A7]
  If Action Subsystem4/2(Out2) -> Subsystem5/1(In1), [B5]
  If Action Subsystem2/3(Out3) -> Subsystem2/1(In1), [C3]
  Constant1/1 -> Subsystem3/2(In2)
  Constant20/1 -> Subsystem5/2(In2)
  Constant4/1 -> Subsystem4/2(In2)
  Constant3/1 -> Subsystem2/2(In2)
  Constant21/1 -> Subsystem6/2(In2)
  Constant39/1 -> Subsystem7/2(In2)
  Constant2/1 -> Subsystem1/2(In2)
  If Action Subsystem1/2(Out2) -> Subsystem1/1(In1), [B2]
  If Action Subsystem5/1(Out1) -> Subsystem6/1(In1), [A6]
  If Action Subsystem3/1(Out1) -> Subsystem4/1(In1), [A4]
  Subsystem1/1(Output) -> Max/2
  Max/1 -> [F_4_Z]
  Subsystem7/1(Output) -> Max/7
  Subsystem6/1(Output) -> Max/6
  Subsystem5/1(Output) -> Max/5
  Subsystem4/1(Output) -> Max/4
  Subsystem2/1(Output) -> Max/3
  Subsystem3/1(Output) -> Max/1

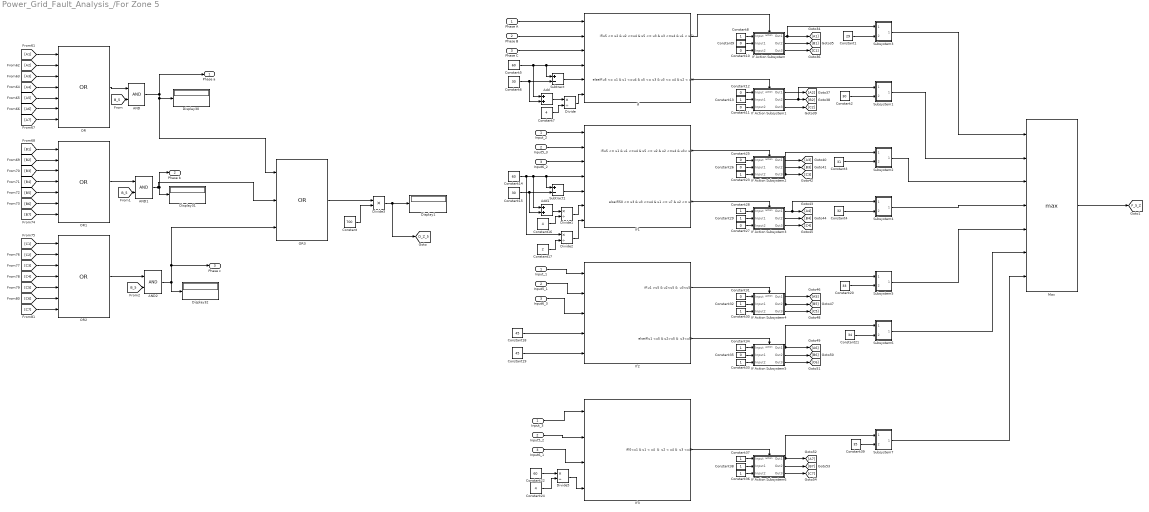
== system Power_Grid_Fault_Analysis_/For Zone 5 ==
  Phase A : Inport
  Phase B : Inport  Port=2
  Phase C : Inport  Port=3
  AND : Logic  IconShape=distinctive  AllPortsSameDT=off  OutDataTypeStr=boolean
  AND1 : Logic  IconShape=distinctive  AllPortsSameDT=off  OutDataTypeStr=boolean
  AND2 : Logic  IconShape=distinctive  AllPortsSameDT=off  OutDataTypeStr=boolean
  Add : Sum
  Add1 : Sum
  Constant : Constant  Value=700
  Constant1 : Constant  Value=29
  Constant{9..12,25..27,31,35} (9 alike) : Constant  Value=0
  Constant{8,13,23,28..30,32..34,36..38} (12 alike) : Constant
  Constant14 : Constant  Value=60
  Constant15 : Constant  Value=30
  Constant16 : Constant  Value=4
  Constant17 : Constant  Value=2
  Constant18 : Constant  Value=45
  Constant19 : Constant  Value=45
  Constant2 : Constant  Value=30
  Constant20 : Constant  Value=33
  Constant21 : Constant  Value=34
  Constant22 : Constant  Value=60
  Constant24 : Constant  Value=4
  Constant3 : Constant  Value=31
  Constant39 : Constant  Value=35
  Constant4 : Constant  Value=32
  Constant5 : Constant  Value=60
  Constant6 : Constant  Value=30
  Constant7 : Constant  Value=4
  Display{1,30..32} (4 alike) : Display
      settings: Decimation=2
  Divide{,1..2,5} (4 alike) : Product  Inputs=*/  SaturateOnIntegerOverflow=on  RndMeth=Zero
  Divide3 : Product  Inputs=**  SaturateOnIntegerOverflow=on  RndMeth=Zero
  If : If  NumInputs=6  IfExpression=u5 <= u2 & u2 <=u4 & u5 <= u3 & u3 <=u4 & u1 < u6  ElseIfExpressions=u5 <= u1 & u1 <=u4 & u5 <= u3 & u3 <= u4 & u2 < u6  ShowElse=off
  If Action Subsystem : Subsystem  TreatAsAtomicUnit=on
  If Action Subsystem1 : Subsystem  TreatAsAtomicUnit=on
  If Action Subsystem2 : Subsystem  TreatAsAtomicUnit=on
  If Action Subsystem3 : Subsystem  TreatAsAtomicUnit=on
  If Action Subsystem4 : Subsystem  TreatAsAtomicUnit=on
  If Action Subsystem5 : Subsystem  TreatAsAtomicUnit=on
  If Action Subsystem6 : Subsystem  TreatAsAtomicUnit=on
  If1 : If  NumInputs=7  IfExpression=u5 <= u1 & u1 <=u4 & u5 <= u2 & u2 <=u4 & u3< u6  ElseIfExpressions=50 <= u3 & u3 <=u4 & u1 <= u7 & u2 <= u7  ShowElse=off
  If2 : If  NumInputs=5  IfExpression="u1 >u5 & u2<u5 &  u3<u5"  ElseIfExpressions="u1 <u5 & u2>u5 &  u3<u5"  ShowElse=off
  If3 : If  NumInputs=4  IfExpression="0<u1 & u1 < u4  &  u2 < u4 &  u3 <u4"  ShowElse=off
  Input5_1 : InportShadow  Port=2
  Input5_2 : InportShadow  Port=2
  Input5_3 : InportShadow  Port=2
  Input6_1 : InportShadow  Port=3
  Input6_2 : InportShadow  Port=3
  Input6_3 : InportShadow  Port=3
  Input_1 : InportShadow
  Input_2 : InportShadow
  Input_3 : InportShadow
  Max : MinMax  Function=max  Inputs=7
  OR : Logic  Operator=OR  Inputs=7  IconShape=distinctive  AllPortsSameDT=off  OutDataTypeStr=boolean
  OR1 : Logic  Operator=OR  Inputs=7  IconShape=distinctive  AllPortsSameDT=off  OutDataTypeStr=boolean
  OR2 : Logic  Operator=OR  Inputs=7  IconShape=distinctive  AllPortsSameDT=off  OutDataTypeStr=boolean
  OR3 : Logic  Operator=OR  Inputs=3  IconShape=distinctive  AllPortsSameDT=off  OutDataTypeStr=boolean
  Subsystem1 : Subsystem
  Subsystem2 : Subsystem
  Subsystem3 : Subsystem
  Subsystem4 : Subsystem
  Subsystem5 : Subsystem
  Subsystem6 : Subsystem
  Subsystem7 : Subsystem
  Subtract : Sum  Inputs=+-
  Subtract1 : Sum  Inputs=+-
  Phase a : Outport
  Phase b : Outport  Port=2
  Phase c : Outport  Port=3
  tag scope: D_Z_5=global, F_5_Z=global
  wires:
  [A1] -> OR/1
  Constant28/1 -> If Action Subsystem3/1(Input)
  Constant23/1 -> If Action Subsystem2/3(Input2)
  Input6_1/1 -> If3/3
  Constant29/1 -> If Action Subsystem3/2(Input1)
  Constant7/1 -> Divide/2
  If Action Subsystem4/1(Out1) -> [A5]
  Constant14/1 -> Divide2/1, Subtract1/1, If1/4, Add1/1
  Input_2/1 -> If1/1
  If Action Subsystem/3(Out3) -> [C1]
  [C1] -> OR2/1
  Constant18/1 -> If2/4
  If Action Subsystem2/1(Out1) -> [A3]
  Divide5/1 -> If3/4
  Add/1 -> Divide/1
  Constant36/1 -> If Action Subsystem6/3(Input2)
  Constant35/1 -> If Action Subsystem5/2(Input1)
  [A6] -> OR/6
  Constant31/1 -> If Action Subsystem4/1(Input)
  If Action Subsystem5/2(Out2) -> [B6]
  [A3] -> OR/3
  [A7] -> OR/7
  Constant13/1 -> If Action Subsystem1/2(Input1)
  If Action Subsystem2/2(Out2) -> [B3]
  If1/1 -> If Action Subsystem2/Action
  [A4] -> OR/4
  Constant32/1 -> If Action Subsystem4/2(Input1)
  Input6_2/1 -> If1/3
  Divide1/1 -> If1/6
  [A2] -> OR/2
  Constant22/1 -> Divide5/1
  Divide2/1 -> If1/7
  Phase C/1 -> If/3
  If Action Subsystem1/3(Out3) -> [C2]
  Constant24/1 -> Divide5/2
  If/2 -> If Action Subsystem1/Action
  Subtract1/1 -> If1/5
  Constant8/1 -> If Action Subsystem/1(Input)
  If Action Subsystem1/1(Out1) -> [A2]
  Constant26/1 -> If Action Subsystem2/2(Input1)
  Constant17/1 -> Divide2/2
  If2/2 -> If Action Subsystem5/Action
  Input_3/1 -> If3/1
  Divide/1 -> If/6
  Constant34/1 -> If Action Subsystem5/1(Input)
  Constant37/1 -> If Action Subsystem6/1(Input)
  If1/2 -> If Action Subsystem3/Action
  If Action Subsystem3/2(Out2) -> [B4]
  [B7] -> OR1/7
  If Action Subsystem6/3(Out3) -> [C7]
  Constant38/1 -> If Action Subsystem6/2(Input1)
  Constant11/1 -> If Action Subsystem1/3(Input2)
  Input6_3/1 -> If2/3
  [B3] -> OR1/3
  [B5] -> OR1/5
  Constant27/1 -> If Action Subsystem3/3(Input2)
  [A5] -> OR/5
  Add1/1 -> Divide1/1
  Constant25/1 -> If Action Subsystem2/1(Input)
  Input5_3/1 -> If1/2
  [C7] -> OR2/7
  [B4] -> OR1/4
  [B1] -> OR1/1
  If Action Subsystem4/3(Out3) -> [C5]
  If/1 -> If Action Subsystem/Action
  Constant16/1 -> Divide1/2
  Constant10/1 -> If Action Subsystem/3(Input2)
  Constant30/1 -> If Action Subsystem4/3(Input2)
  If Action Subsystem5/3(Out3) -> [C6]
  If3/1 -> If Action Subsystem6/Action
  [B6] -> OR1/6
  Constant6/1 -> Add/2, Subtract/2
  [C2] -> OR2/2
  Constant33/1 -> If Action Subsystem5/3(Input2)
  [B2] -> OR1/2
  Phase A/1 -> If/1
  Constant9/1 -> If Action Subsystem/2(Input1)
  [C5] -> OR2/5
  If Action Subsystem3/3(Out3) -> [C4]
  Constant15/1 -> Subtract1/2, Add1/2
  Phase B/1 -> If/2
  Input_1/1 -> If2/1
  Input5_1/1 -> If2/2
  [C6] -> OR2/6
  If Action Subsystem/2(Out2) -> [B1]
  [C4] -> OR2/4
  Constant19/1 -> If2/5
  [C3] -> OR2/3
  Constant5/1 -> Add/1, Subtract/1, If/4
  If2/1 -> If Action Subsystem4/Action
  Subtract/1 -> If/5
  If Action Subsystem6/2(Out2) -> [B7]
  Input5_2/1 -> If3/2
  Constant12/1 -> If Action Subsystem1/1(Input)
  Divide3/1 -> [D_Z_5], Display1/1
  Constant/1 -> Divide3/2
  OR/1 -> AND/1
  OR3/1 -> Divide3/1
  AND/1 -> Phase a/1, OR3/1, Display30/1
  [B_5] -> AND/2
  [B_5] -> AND1/2
  OR1/1 -> AND1/1
  AND1/1 -> OR3/2, Phase b/1, Display31/1
  [B_5] -> AND2/2
  OR2/1 -> AND2/1
  AND2/1 -> OR3/3, Phase c/1, Display32/1
  If Action Subsystem/1(Out1) -> Subsystem3/1(In1), [A1]
  If Action Subsystem6/1(Out1) -> Subsystem7/1(In1), [A7]
  If Action Subsystem4/2(Out2) -> Subsystem5/1(In1), [B5]
  If Action Subsystem2/3(Out3) -> Subsystem2/1(In1), [C3]
  Constant1/1 -> Subsystem3/2(In2)
  Constant20/1 -> Subsystem5/2(In2)
  Constant4/1 -> Subsystem4/2(In2)
  Constant3/1 -> Subsystem2/2(In2)
  Constant21/1 -> Subsystem6/2(In2)
  Constant39/1 -> Subsystem7/2(In2)
  Constant2/1 -> Subsystem1/2(In2)
  If Action Subsystem1/2(Out2) -> Subsystem1/1(In1), [B2]
  If Action Subsystem5/1(Out1) -> Subsystem6/1(In1), [A6]
  If Action Subsystem3/1(Out1) -> Subsystem4/1(In1), [A4]
  Subsystem1/1(Output) -> Max/2
  Max/1 -> [F_5_Z]
  Subsystem7/1(Output) -> Max/7
  Subsystem6/1(Output) -> Max/6
  Subsystem5/1(Output) -> Max/5
  Subsystem4/1(Output) -> Max/4
  Subsystem2/1(Output) -> Max/3
  Subsystem3/1(Output) -> Max/1

== system Power_Grid_Fault_Analysis_/If Action Subsystem ==
  Input : Inport
  Action Port : ActionPort  ActionPortLabel=|
      | if(u1==1|u1==8|u1==15|u1==22|u1==29
      | )
  Out1 : Outport
  wires:
  Input/1 -> Out1/1

== system Power_Grid_Fault_Analysis_/If Action Subsystem1 ==
  Input : Inport
  Action Port : ActionPort  ActionPortLabel=|
      | elseif(u1==2|u1==9|u1==16|u1==23|u1==30
      | )
  Out1 : Outport
  wires:
  Input/1 -> Out1/1

== system Power_Grid_Fault_Analysis_/If Action Subsystem2 ==
  Input : Inport
  Action Port : ActionPort  ActionPortLabel=|
      | if(u1==3|u1==10|u1==17|u1==24|u1==31
      | )
  Out1 : Outport
  wires:
  Input/1 -> Out1/1

== system Power_Grid_Fault_Analysis_/If Action Subsystem3 ==
  Input : Inport
  Action Port : ActionPort  ActionPortLabel=|
      | elseif(u1==4|u1==11|u1==18|u1==25|u1==32
      | )
  Out1 : Outport
  wires:
  Input/1 -> Out1/1

== system Power_Grid_Fault_Analysis_/If Action Subsystem4 ==
  Input : Inport
  Action Port : ActionPort  ActionPortLabel=|
      | if(u1==5|u1==12|u1==19|u1==26|u1==33
      | )
  Out1 : Outport
  wires:
  Input/1 -> Out1/1

== system Power_Grid_Fault_Analysis_/If Action Subsystem5 ==
  Input : Inport
  Action Port : ActionPort  ActionPortLabel=|
      | elseif(u1==6|u1==13|u1==20|u1==27|u1==34
      | )
  Out1 : Outport
  wires:
  Input/1 -> Out1/1

== system Power_Grid_Fault_Analysis_/If Action Subsystem6 ==
  Input : Inport
  Action Port : ActionPort  ActionPortLabel=|
      | if(u1==7|u1==14|u1==21|u1==28|u1==35
      | )
  Out1 : Outport
  wires:
  Input/1 -> Out1/1

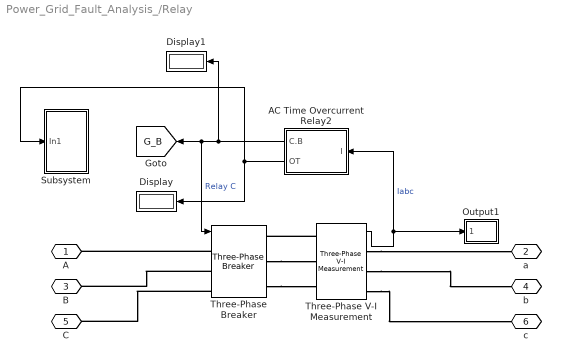
== system Power_Grid_Fault_Analysis_/Relay  ==
  AC Time Overcurrent Relay2 : Subsystem  mask(AC Time Overcurrent Relay Block){tcpopup=Definite Minimum Time, k=0, alpha=0.02, B=0, PS=100%, TMS=0.1, TDS=5, CTpri=300, CTsec=5, Freq=60, RMSInit=0}
      mask prompts: tcpopup "Trip Characteristic"; PS "Plug Setting (PS) / Low-set (I >)"; TMS "Time Multiplier Setting (TMS)"; TDS "Time Delay Setting (TDS) in sec"; CTpri "Current Transformer Primary (A)"; CTsec "Current Transformer Secondary (A)"; Freq "Fundamental frequency (Hz):"; RMSInit "Initial RMS value:"
      mask help:
      | AC Time Overcurrent Relay Block developed by Dr Rodney Tan
      | Version 1.0 (Jun 2016)
      |
      | AC Time Overcurrent Relay (ANSI/IEEE C37.2 device number 51) that operates when the current exceeds a predetermined value.
      |
      | This relay operates with either a Definite Minimum Time (DMT) or Inverse Definite Minimum Time (IDMT) characteristic.
      |
      | This relay support both IEC 60255 Standard and IEEE Standard C37.112-1996 IDMT trip characteristic.
      mask Help:
      | <b><u>Block Setting</u></b>
      | <b>Trip Characteristic</b>
      | Relay operation mode selection of Definite Minimum Time (DMT), IEC 60255 Standard or IEEE Standard C37.112-1996 Inverse Definite Minimum Time (IDMT).
      | 
      | <b>Plug-Setting(PS) / Low-set (I >)</b>
      | Specify relay pick-up current based on current transformer rating ranging from 25% to 200% with 25% step interval.
      | 
      | <b>Time Multiplier Setting (TMS)</b>
      | Specify time delay multiplier ranging from 0.05 to 1.0 for IDMT relay operation. This setting will be disabled DMT relay operation mode.
      | 
      | <b>Plot Curve Button</b>
      | Plot current Inverse Definite Minimum Time trip curve.
      | 
      | <b>Time Delay Setting (TDS)</b>
      | Specify time delay ranging from 0.05sec to 99sec for Definite Minimum Time relay operation. This setting will be disabled in IDMT relay operation mode.
      | 
      | <b>Current Transformer Primary (A)</b>
      | Specify current transformer primary in Ampere.
      | 
      | <b>Current Transformer Secondary (A)</b>
      | Specify current transformer secondary in Ampere.
      | 
      | <b>Fundamental Frequency (Hz)</b>
      | Specify the RMS current measurement fundamental frequency, in hertz, of the input signal.
      | 
      | <b>Initial RMS Value</b>
      | Specify the RMS current measurement initial RMS value of the output signal.
      | 
      | <b><u>Block Input Output</u></b>
      | <b>I</b>
      | Current input to the AC time overcurrent relay
      | 
      | <b>trip</b>
      | Trip control signal output (1-0), commonly connected to circuit breaker
      | 
      | <b>OT</b>
      | Relay operating time output
      mask TypeOptions tcpopup: Definite Minimum Time | IEC Standard Inverse | IEC Very Inverse | IEC Long Time Inverse | IEC Extremely Inverse | IEC Ultra Inverse | IEEE Moderately Inverse | IEEE Very Inverse | IEEE Extremely Inverse
      mask Callback tcpopup:
      | switch(get_param(gcb,'tcpopup'))
      |     case 'IEC Standard Inverse'
      |         set_param(gcb,'k','0.14');
      |         set_param(gcb,'alpha','0.02');
      |         set_param(gcb,'B','0');
      |         set_param(gcb,'MaskEnables',{'on','off','off','off',...
      |                   'on','on','off','on','on','on','on'});
      |     case 'IEC Very Inverse'
      |         set_param(gcb,'k','13.5');
      |         set_param(gcb,'alpha','1');
      |         set_param(gcb,'B','0');
      |         set_param(gcb,'MaskEnables',{'on','off','off','off',...
      |                   'on','on','off','on','on','on','on'});
      |     case 'IEC Long Time Inverse'
      |         set_param(gcb,'k','120');
      |         set_param(gcb,'alpha','1');
      |         set_param(gcb,'B','0');
      |         set_param(gcb,'MaskEnables',{'on','off','off','off',...
      |                   'on','on','off','on','on','on','on'});
      |     case 'IEC Extremely Inverse'
      |         set_param(gcb,'k','80');
      |         set_param(gcb,'alpha','2');
      |         set_param(gcb,'B','0');
      |         set_param(gcb,'MaskEnables',{'on','off','off','off',...
      |                   'on','on','off','on','on','on','on'});
      |     case 'IEC Ultra Inverse'
      |         set_param(gcb,'k','315.2');
      |         set_param(gcb,'alpha','2.5');
      |         set_param(gcb,'B','0');
      |         set_param(gcb,'MaskEnables',{'on','off','off','off',...
      |                   'on','on','off','on','on','on','on'});
      |     case 'IEEE Moderately Inverse'
      |         set_param(gcb,'k','0.0515');
      |         set_param(gcb,'alpha','0.02');
      |         set_param(gcb,'B','0.114');
      |         set_param(gcb,'MaskEnables',{'on','off','off','off',...
      |                   'on','on','off','on','on','on','on'});
      |     case 'IEEE Very Inverse'
      |         set_param(gcb,'k','19.61');
      |         set_param(gcb,'alpha','2');
      |         set_param(gcb,'B','0.491');
      |         set_param(gcb,'MaskEnables',{'on','off','off','off',...
      |                   'on','on','off','on','on','on','on'});
      |     case 'IEEE Extremely Inverse'
      |         set_param(gcb,'k','28.2');
      |         set_param(gcb,'alpha','2');
      |         set_param(gcb,'B','0.1217');
      |         set_param(gcb,'MaskEnables',{'on','off','off','off',...
      |                   'on','on','off','on','on','on','on'});
      |     otherwise
      |         set_param(gcb,'k','0');
      |         set_param(gcb,'MaskEnables',{'on','off','off','off',...
      |                   'on','off','on','on','on','on','on'});
      | end
      mask TypeOptions PS: 25% | 50% | 75% | 100% | 125% | 150% | 175% | 200%
      mask TypeOptions TMS: 0.05 | 0.1 | 0.15 | 0.2 | 0.25 | 0.3 | 0.35 | 0.4 | 0.45 | 0.5 | 0.55 | 0.6 | 0.65 | 0.7 | 0.75 | 0.8 | 0.85 | 0.9 | 0.95 | 1.0
      mask Callback TDS:
      | TDS = str2double(get_param(gcb,'TDS'));
      | if (TDS > 99)||(TDS < 0.05)||isnan(TDS)
      |     msgbox('TDS must be in the range of 0.05-99 sec',...
      |     'Invalid Value !','error');
      |     set_param(gcb,'TDS','0.1');
      | end
      mask TypeOptions Freq: Irms/Freq
      mask TypeOptions RMSInit: Irms/RMSInit
      mask DialogControl Container2 Prompt: Relay Setting
      mask DialogControl plotbutton Prompt: Plot Curve
      mask DialogControl plotbutton Callback:
      | % Plotting IDMT Curve
      | TMS = str2num(get_param(gcb,'TMS'));
      | k = str2num(get_param(gcb,'k'));
      | alpha = str2num(get_param(gcb,'alpha'));
      | B = str2num(get_param(gcb,'B'));
      | I = 1:20;
      | td = ((k./((I.^alpha)-1))+B)*TMS;
      | loglog(td);
      | set(gcf, 'Position', [200 150 300 500]);
      | switch(get_param(gcb,'tcpopup'))
      |     case 'IEC Standard Inverse'
      |         title('IEC Standard Inverse');
      |         set(gca, 'YTick', (1:10));
      |         ylim([0.1 10]);
      |     case 'IEC Very Inverse'
      |         title('IEC Very Inverse');
      |         set(gca, 'YTick', (1:2:15));
      |         ylim([0.01 15]);
      |     case 'IEC Long Time Inverse'
      |         title('IEC Long Time Inverse');
      |         set(gca, 'YTick', (0:20:120));
      |         ylim([0.1 120]);
      |     case 'IEC Extremely Inverse'
      |         title('IEC Extremely Inverse');
      |         set(gca, 'YTick', (0:5:30));
      |         ylim([0.01 30]);
      |     case 'IEC Ultra Inverse'
      |         title('IEC Ultra Inverse');
      |         set(gca, 'YTick', (0:20:100));
      |         ylim([0.01 100]);
      |     case 'IEEE Moderately Inverse'
      |         title('IEEE Moderately Inverse');
      |         set(gca, 'YTick', (1:5));
      |         ylim([0.01 5]);
      |     case 'IEEE Very Inverse'
      |         title('IEEE Very Inverse');
      |         set(gca, 'YTick', (1:10));
      |         ylim([0.01 10]);
      |     case 'IEEE Extremely Inverse'
      |         title('IEEE Extremely Inverse');
      |         set(gca, 'YTick', (1:10));
      |         ylim([0.01 10]);
      | end
      | 
      | set(gca, 'XTick', [1:10 20]);
      | xlim([1 30]);
      | xlabel('Current (Multiples of Plug Setting)');
      | ylabel('Operating Time (sec)');
      | grid on;
      mask DialogControl Container3 Prompt: Current Transformer Setting
      mask DialogControl RMS Prompt: RMS Current Measurement
      mask Display:
      | disp('(51)');
      | port_label('input', 1, 'I');
      | port_label('output', 1, 'trip');
      | port_label('output', 2, 'OT');
  Display : Display
  Display1 : Display
  Output1 : Subsystem
  Subsystem : Subsystem
  Three-Phase V-I Measurement : powerlib/Measurements/Three-Phase V-I Measurement  VoltageMeasurement=no  SetLabelV=off  LabelV=Vabc  Vpu=off  VpuLL=off  CurrentMeasurement=yes  SetLabelI=off  LabelI=Iabc  Ipu=off  Pbase=100e6  Vbase=500e3  OutputType=Complex  PhasorSimulation=off  PSBequivalent=0
      settings: SourceProductName=Simscape Electrical
  Three-Phase Breaker : powerlib/Elements/Three-Phase Breaker  InitialState=closed  SwitchA=on  SwitchB=on  SwitchC=on  SwitchTimes="[1/60  5/60]"  External=on  BreakerResistance=0.001  SnubberResistance=1e6  SnubberCapacitance=inf  Measurements=None
      settings: SourceProductName=Simscape Electrical
  A : PMIOPort  Side=Left
  a : PMIOPort  Port=2  Side=Right
  B : PMIOPort  Port=3  Side=Left
  b : PMIOPort  Port=4  Side=Right
  C : PMIOPort  Port=5  Side=Left
  c : PMIOPort  Port=6  Side=Right
  tag scope: G_B=global
  wires:
  Three-Phase V-I Measurement/1 -> Output1/1(Signal), AC Time Overcurrent Relay2/1(I)  "Iabc"
  AC Time Overcurrent Relay2/2(OT) -> Subsystem/1(In1), Display/1
  AC Time Overcurrent Relay2/1(C.B) -> Display1/1, [G_B], Three-Phase Breaker/1  "Relay C"
  connections:
  Three-Phase Breaker/RConn2 -- Three-Phase V-I Measurement/LConn2
  Three-Phase V-I Measurement/RConn2 -- b/RConn1
  Three-Phase V-I Measurement/LConn1 -- Three-Phase Breaker/RConn1
  Three-Phase Breaker/LConn2 -- B/RConn1
  Three-Phase V-I Measurement/RConn1 -- a/RConn1
  Three-Phase Breaker/RConn3 -- Three-Phase V-I Measurement/LConn3
  Three-Phase Breaker/LConn3 -- C/RConn1
  Three-Phase V-I Measurement/RConn3 -- c/RConn1
  Three-Phase Breaker/LConn1 -- A/RConn1
